simulink model "ex1"  (R2023a)
settings: Solver=FixedStepAuto  StartTime=0.0  StopTime=3600*24*100  FixedStep=100  RelTol=1e-3
values from neighbouring files (symbols this model uses):
  mu = astroConstants(13)    [Lab_1.m]    (also in Lab_2.m)
  r = ECI_coord(tspan,r_0,v_0,mu)    [Lab_1.m]    (also in car2ECI.m = y(:, 1:3); eci2ra.m = r'; kep2car.m = [r; (R*r_pf)']; keplerian_orbit_ode.m = y(:, 1:3))
  v = y(:, 4:6)    [car2ECI.m]    (also in kep2car.m = [v; (R*v_pf)']; keplerian_orbit_ode.m; ode_2bp.m = y(4:6); sol_errors.m = v')
settings Model: Creator=francesconuzzo  LastModifiedBy=francesconuzzo
settings SolverCC: EnableFixedStepZeroCrossing=on

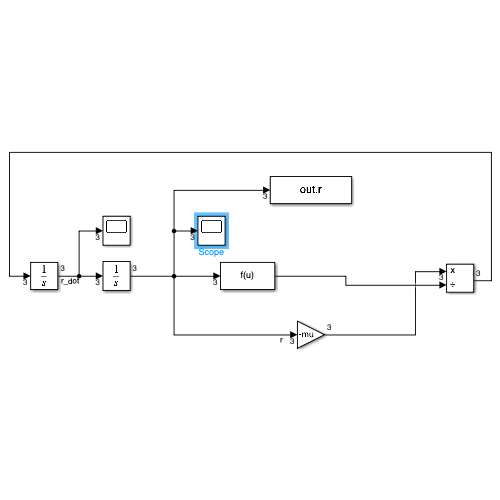
[thumbnail: Simulink's stored preview of the top-level diagram]
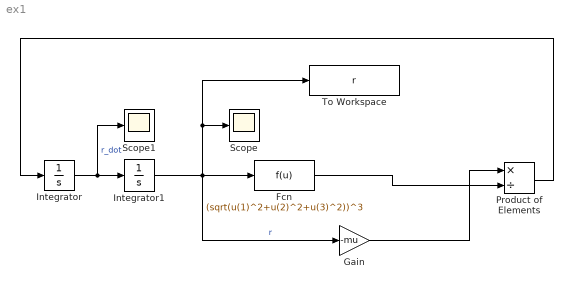
== system ex1 ==
  Fcn : Fcn  Expr=(sqrt(u(1)^2+u(2)^2+u(3)^2))^3
  Gain : Gain  Gain=-mu
  Integrator : Integrator  InitialCondition=v
  Integrator1 : Integrator  InitialCondition=r
  Product of Elements : Product  Inputs=*/
  Scope : Scope
  Scope1 : Scope
  To Workspace : ToWorkspace  VariableName=r  SampleTime=-1
  wires:
  Integrator/1 -> Scope1/1, Integrator1/1  "r_dot"
  Integrator1/1 -> Fcn/1, Gain/1, To Workspace/1, Scope/1  "r"
  Fcn/1 -> Product of Elements/2
  Gain/1 -> Product of Elements/1
  Product of Elements/1 -> Integrator/1
